simulink model "PMSM_simulink"  (R2014b)
settings: Solver=ode23t  StartTime=0.0  StopTime=0.1  RelTol=1e-3
libraries: powerlib_extras x3, powerlib x1
settings Model: Creator=Administrator  LastModifiedBy=Lei
settings DataIOCC: SignalLoggingSaveFormat=ModelDataLogs
settings OptimizationCC: ExpressionDepthLimit=2147483647  InitFltsAndDblsToZero=on
settings DebuggingCC: SaveWithParameterizedLinksMsg=none  UnderspecifiedInitializationDetection=Classic  MergeDetectMultiDrivingBlocksExec=none  FcnCallInpInsideContextMsg=UseLocalSettings  StateNameClashWarn=warning  StrictBusMsg=Warning
settings GRTTargetCC: TargetFcnLib=ansi_tfl_tmw.mat  CombineOutputUpdateFcns=off  GRTInterface=on

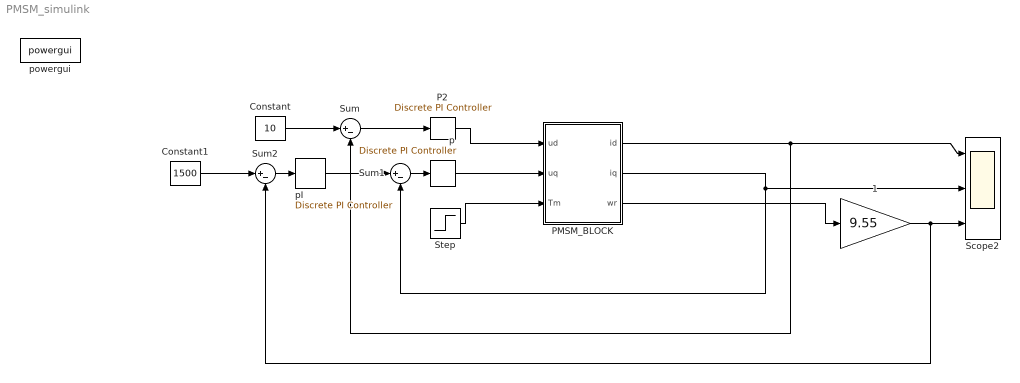
== system PMSM_simulink ==
  1 : Gain  Gain=9.55
  Constant : Constant  Value=10
  Constant1 : Constant  Value=1500
  "P2 " : powerlib_extras/Discrete  Control Blocks/Discrete PI Controller  Kp=21.25  Ki=7187.5  Par_Limits=[250 -250]  Init=0  Ts=50e-6
  PMSM_BLOCK : Subsystem  mask{P=4, Phi=0.175, Ld=8.5e-3, Lq=8.5e-3, R=2.875, F=0.8e-3, J=1e-3}
  Scope2 : Scope  NumInputPorts=3
      settings: YMin=1575~-5~-5  YMax=1685~5~5
  Step : Step  Time=0.1  After=10  SampleTime=0
  Sum : Sum  Inputs=|+-
  Sum1 : Sum  Inputs=|+-
  Sum2 : Sum  Inputs=|+-
  p : powerlib_extras/Discrete  Control Blocks/Discrete PI Controller  Kp=21.25  Ki=7187.5  Par_Limits=[300 -200]  Init=0  Ts=50e-6
  "pI " : powerlib_extras/Discrete  Control Blocks/Discrete PI Controller  Kp=0.06  Ki=1  Par_Limits=[300 -300]  Init=0  Ts=50e-6
  powergui : powerlib/powergui  SimulationMode=Continuous  SolverType=Tustin/Backward Euler (TBE)  SampleTime=50e-6  frequency=60  SPID=off  DisableSnubberDevices=off  DisableRonSwitches=off  DisableVfSwitches=off  SwTol=0  DisplayEquations=off  Interpol=off  methode=off  Ts=0  frequencyindice=0  Pbase=100e6  ErrMax=1e-4  Iterations=50  UnitsV=kV  UnitsW=MW  FunctionMessages=off  echomessages=off  HookPort=off  EnableUseOfTLC=off  x0status=blocks  RestoreLinks=warning  ResistiveCurrentMeasurement=off  Frange=[0:2:500]  Ylog=off  Xlog=on  ShowGrid=off  save=off  variable=ZData  structure=0  ZoomFFT=off  StartTime=0.0  cycles=1  DisplayStyle=1  fundamental=60  FreqAxis=off  MaxFrequency=1000  frequencyindicesteady=1  RmsSteady=1  display=off
  wires:
  Sum/1 -> "P2 "/1
  Sum1/1 -> p/1
  "pI "/1 -> Sum1/1
  Constant/1 -> Sum/1
  Sum2/1 -> "pI "/1
  1/1 -> Sum2/2, Scope2/3
  Constant1/1 -> Sum2/1
  PMSM_BLOCK/1(id) -> Sum/2, Scope2/1
  PMSM_BLOCK/2(iq) -> Sum1/2, Scope2/2
  p/1 -> PMSM_BLOCK/2(uq)
  "P2 "/1 -> PMSM_BLOCK/1(ud)
  PMSM_BLOCK/3(wr) -> 1/1
  Step/1 -> PMSM_BLOCK/3(Tm)

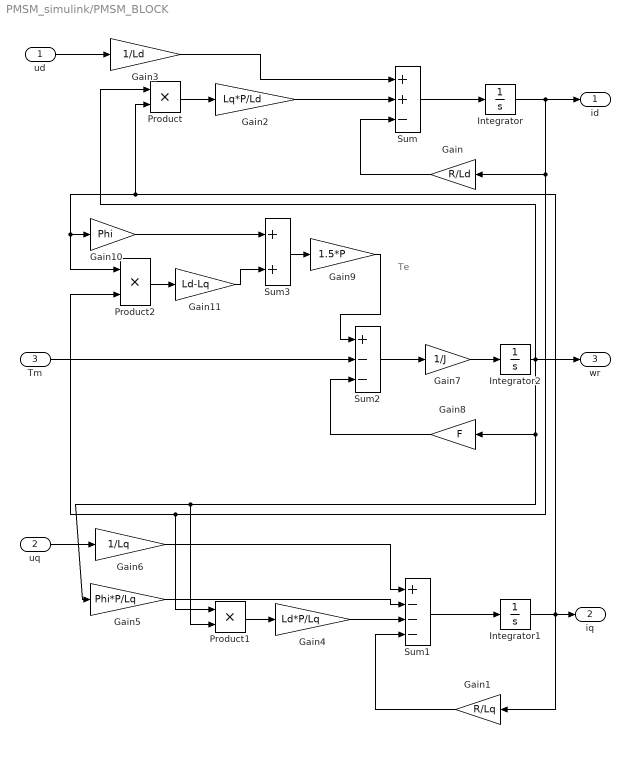
== system PMSM_simulink/PMSM_BLOCK ==
  note: Te
  ud : Inport
  uq : Inport  Port=2
  Tm : Inport  Port=3
  Gain : Gain  Gain=R/Ld
  Gain1 : Gain  Gain=R/Lq
  Gain10 : Gain  Gain=Phi
  Gain11 : Gain  Gain=Ld-Lq
  Gain2 : Gain  Gain=Lq*P/Ld
  Gain3 : Gain  Gain=1/Ld
  Gain4 : Gain  Gain=Ld*P/Lq
  Gain5 : Gain  Gain=Phi*P/Lq
  Gain6 : Gain  Gain=1/Lq
  Gain7 : Gain  Gain=1/J
  Gain8 : Gain  Gain=F
  Gain9 : Gain  Gain=1.5*P
  Integrator : Integrator
  Integrator1 : Integrator
  Integrator2 : Integrator
  Product : Product  RndMeth=Zero
  Product1 : Product  RndMeth=Zero
  Product2 : Product  RndMeth=Zero
  Sum : Sum  Inputs=++-
  Sum1 : Sum  Inputs=+---
  Sum2 : Sum  Inputs=+--
  Sum3 : Sum
  id : Outport
  iq : Outport  Port=2
  wr : Outport  Port=3
  wires:
  Gain9/1 -> Sum2/1
  Sum3/1 -> Gain9/1
  Gain11/1 -> Sum3/2
  Product2/1 -> Gain11/1
  Gain10/1 -> Sum3/1
  Tm/1 -> Sum2/2
  Gain8/1 -> Sum2/3
  Sum2/1 -> Gain7/1
  Gain7/1 -> Integrator2/1
  Integrator2/1 -> Gain5/1, Product1/2, Gain8/1, Product/1, wr/1
  Gain6/1 -> Sum1/1
  uq/1 -> Gain6/1
  Gain5/1 -> Sum1/2
  Product1/1 -> Gain4/1
  Product/1 -> Gain2/1
  Gain4/1 -> Sum1/3
  Gain1/1 -> Sum1/4
  Sum1/1 -> Integrator1/1
  Integrator1/1 -> Product2/1, Gain10/1, Product/2, Gain1/1, iq/1
  Gain3/1 -> Sum/1
  ud/1 -> Gain3/1
  Gain2/1 -> Sum/2
  Gain/1 -> Sum/3
  Sum/1 -> Integrator/1
  Integrator/1 -> Product2/2, Product1/1, Gain/1, id/1
